simulink model "lab3"  (R2021a)
settings: Solver=VariableStepAuto  StartTime=0.0  StopTime=10.0  MaxStep=1e-3  RelTol=1e-3
libraries: simulink x7
settings Model: Creator=reemb  LastModifiedBy=reemb

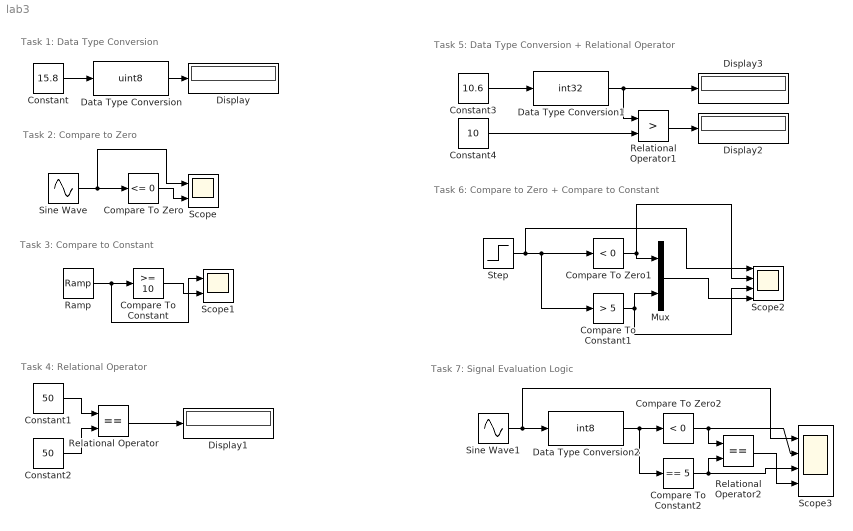
== system lab3 ==
  note: Task 7: Signal Evaluation Logic
  note: Task 6: Compare to Zero + Compare to Constant
  note: Task 5: Data Type Conversion + Relational Operator
  note: Task 4: Relational Operator
  note: Task 3: Compare to Constant
  note: Task 2: Compare to Zero
  note: Task 1: Data Type Conversion
  Compare To Constant : simulink/Logic and Bit Operations/Compare To Constant  relop=>=  const=10  OutDataTypeStr=boolean
  Compare To Constant1 : simulink/Logic and Bit Operations/Compare To Constant  relop=>  const=5  OutDataTypeStr=boolean
  Compare To Constant2 : simulink/Logic and Bit Operations/Compare To Constant  relop===  const=5  OutDataTypeStr=boolean
  Compare To Zero : simulink/Logic and Bit Operations/Compare To Zero  relop=<=  OutDataTypeStr=boolean
  Compare To Zero1 : simulink/Logic and Bit Operations/Compare To Zero  relop=<  OutDataTypeStr=boolean
  Compare To Zero2 : simulink/Logic and Bit Operations/Compare To Zero  relop=<  OutDataTypeStr=boolean
  Constant : Constant  Value=15.8
  Constant1 : Constant  Value=50
  Constant2 : Constant  Value=50
  Constant3 : Constant  Value=10.6
  Constant4 : Constant  Value=10
  Data Type Conversion : DataTypeConversion  OutDataTypeStr=uint8  RndMeth=Round
  Data Type Conversion1 : DataTypeConversion  OutDataTypeStr=int32  RndMeth=Round
  Data Type Conversion2 : DataTypeConversion  OutDataTypeStr=int8  RndMeth=Round
  Display{,1..3} (4 alike) : Display
  Mux : Mux  Inputs=2
  Ramp : simulink/Sources/Ramp  slope=2  start=0  InitialOutput=0
  Relational Operator : RelationalOperator  Operator===  OutDataTypeStr=boolean  RndMeth=Simplest
  Relational Operator1 : RelationalOperator  Operator=>  OutDataTypeStr=boolean  RndMeth=Simplest
  Relational Operator2 : RelationalOperator  Operator===  OutDataTypeStr=boolean  RndMeth=Simplest
  Scope : Scope  NumInputPorts=2
  Scope1 : Scope  NumInputPorts=2
  Scope2 : Scope  NumInputPorts=4
  Scope3 : Scope  NumInputPorts=4
  Sine Wave : Sin  Amplitude=5  SampleTime=0
  Sine Wave1 : Sin  Amplitude=10  SampleTime=0
  Step : Step  Time=5  Before=-10  After=10  SampleTime=0
  wires:
  Constant/1 -> Data Type Conversion/1
  Data Type Conversion/1 -> Display/1
  Sine Wave/1 -> Scope/1, Compare To Zero/1
  Compare To Zero/1 -> Scope/2
  Ramp/1 -> Scope1/1, Compare To Constant/1
  Compare To Constant/1 -> Scope1/2
  Constant1/1 -> Relational Operator/1
  Constant2/1 -> Relational Operator/2
  Relational Operator/1 -> Display1/1
  Constant3/1 -> Data Type Conversion1/1
  Constant4/1 -> Relational Operator1/2
  Data Type Conversion1/1 -> Relational Operator1/1, Display3/1
  Relational Operator1/1 -> Display2/1
  Step/1 -> Scope2/1, Compare To Constant1/1, Compare To Zero1/1
  Compare To Zero1/1 -> Scope2/2, Mux/1
  Compare To Constant1/1 -> Mux/2, Scope2/3
  Mux/1 -> Scope2/4
  Sine Wave1/1 -> Scope3/1, Data Type Conversion2/1
  Data Type Conversion2/1 -> Compare To Constant2/1, Compare To Zero2/1
  Compare To Zero2/1 -> Scope3/2, Relational Operator2/1
  Compare To Constant2/1 -> Scope3/3, Relational Operator2/2
  Relational Operator2/1 -> Scope3/4
